simulink model "test_integration"  (R2022b)
settings: Solver=FixedStepAuto  StartTime=0.0  StopTime=240  FixedStep=0.1  RelTol=1e-3
(part 2 of 2)

== stateflow chart test_integration/Test Assessment Block ==
  state IncreasePower
    state Init
      state Verify_IP_Init
        verify(alert_led==0 && led==0 && onoff_led==0);
        settings: description=|
            | Inizializzazione.
            | Tutti i led sono spenti.
      state Verify_IP_TurnON
        verify(alert_led==0 && led==0 && onoff_led==1);
        settings: description=|
            | Accensione dispositivo.
            | Il led di accensione è acceso.
      state Verify_IP_IncreasePower300W
        verify(alert_led==0 && led==0 && onoff_led==1);
        settings: description=|
            | Richiesta di aumento potenza.
            | Il led di accensione è acceso.
      state Verify_IP_Wait300W
        verify(alert_led==0 && led==0 && onoff_led==1);
        settings: description=|
            | Attesa passaggio di potenza.
            | Il led di accensione è acceso.
      state Verify_IP_Set300W
        verify(alert_led==0 && led==1 && onoff_led==1)
        settings: description=|
            | Conferma della nuova potenza.
            | Il led di accensione è acceso ed il led giallo di attivazione sta blinkando con periodo di 2 s.
      state Verify_IP_IncreasePower500W
        verify(alert_led==0 && led==1 && onoff_led==1);
        settings: description=|
            | Richiesta di ulteriore incremento della potenza.
            | Il led di accensione è acceso ed il led giallo di attivazione sta blinkando con periodo di 2 s.
      state Verify_IP_Wait500W
        settings: description=Attesa del passaggio di potenza.
        state Verify__IP_Wait500W_1
          verify(alert_led==0 && led==1 && onoff_led==1);
          settings: description=led giallo di attivazione on
        state Verify_IP_Wait500W_2
          verify(alert_led==0 && led==0 && onoff_led==1);
          settings: description=led giallo di attivazione off
        state Verify_IP_Wait500W_3
          verify(alert_led==0 && led==1 && onoff_led==1);
          settings: description=|
              | led giallo di attivazione on
              | led giallo di attivazione off
        state Verify_IP_Wait500W_4
          verify(alert_led==0 && led==0 && onoff_led==1);
        (default) -> Verify__IP_Wait500W_1
        Verify__IP_Wait500W_1 -> Verify_IP_Wait500W_2 : [
            | after(2-(1+2*SamplePeriod),sec)
            | ]
        Verify_IP_Wait500W_2 -> Verify_IP_Wait500W_3 : [
            | after(2,sec)
            | ]
        Verify_IP_Wait500W_3 -> Verify_IP_Wait500W_4 : [
            | after(2,sec)
            | ]
      state Verify_IP_Set500W
        verify(alert_led==0 && led==0 && onoff_led==1)
        settings: description=|
            | Conferma della nuova potenza.
            | Il led di accensione è acceso ed il led giallo di attivazione sta blinkando con periodo di 1 s.
      state Init_1
      (default) -> (junction 144)
      IncreasePower.Init -> (junction 144)
      (junction 144) -> (junction 145) [order 1] : [Active_Step_In == ActiveStepInt.IP_Init
          | ]
      (junction 145) -> Verify_IP_Init [order 1] : [~in(IncreasePower.Init.Verify_IP_Init)]
      (junction 144) -> (junction 154) [order 2]
      (junction 145) -> (junction 148) [order 2]
      (junction 154) -> (junction 155) [order 1] : [Active_Step_In == ActiveStepInt.IP_TurnON
          | ]
      (junction 155) -> Verify_IP_TurnON [order 1] : [~in(IncreasePower.Init.Verify_IP_TurnON)]
      (junction 154) -> (junction 162) [order 2]
      (junction 155) -> (junction 158) [order 2]
      (junction 162) -> (junction 163) [order 1] : [Active_Step_In == ActiveStepInt.IP_IncreasePower300W
          | ]
      (junction 163) -> Verify_IP_IncreasePower300W [order 1] : [~in(IncreasePower.Init.Verify_IP_IncreasePower300W)]
      (junction 162) -> (junction 170) [order 2]
      (junction 163) -> (junction 166) [order 2]
      (junction 170) -> (junction 171) [order 1] : [Active_Step_In == ActiveStepInt.IP_Wait300W
          | ]
      (junction 171) -> Verify_IP_Wait300W [order 1] : [~in(IncreasePower.Init.Verify_IP_Wait300W)]
      (junction 170) -> (junction 178) [order 2]
      (junction 171) -> (junction 174) [order 2]
      (junction 178) -> (junction 179) [order 1] : [Active_Step_In == ActiveStepInt.IP_Set300W
          | ]
      (junction 179) -> Verify_IP_Set300W [order 1] : [~in(IncreasePower.Init.Verify_IP_Set300W)]
      (junction 178) -> (junction 186) [order 2]
      (junction 179) -> (junction 182) [order 2]
      (junction 186) -> (junction 187) [order 1] : [Active_Step_In == ActiveStepInt.IP_IncreasePower500W
          | ]
      (junction 187) -> Verify_IP_IncreasePower500W [order 1] : [~in(IncreasePower.Init.Verify_IP_IncreasePower500W)]
      (junction 186) -> (junction 195) [order 2]
      (junction 187) -> (junction 190) [order 2]
      (junction 195) -> (junction 196) [order 1] : [Active_Step_In == ActiveStepInt.IP_Wait500W
          | ]
      (junction 196) -> Verify_IP_Wait500W [order 1] : [~in(IncreasePower.Init.Verify_IP_Wait500W)]
      (junction 195) -> (junction 203) [order 2]
      (junction 196) -> (junction 199) [order 2]
      (junction 203) -> (junction 204) [order 1] : [Active_Step_In == ActiveStepInt.IP_Set500W
          | ]
      (junction 204) -> Verify_IP_Set500W [order 1] : [~in(IncreasePower.Init.Verify_IP_Set500W)]
      (junction 203) -> (junction 211) [order 2]
      (junction 204) -> (junction 207) [order 2]
      (junction 211) -> (junction 212)
      (junction 212) -> IncreasePower.Init.Init_1 [order 1] : [~in(IncreasePower.Init.Init_1)]
      (junction 212) -> (junction 215) [order 2]
    (default) -> IncreasePower.Init
  state DecreasePower
    state Init
      state Verify_DP_Init
        verify(alert_led==0 && led==0 && onoff_led==0);
        settings: description=|
            | Inizializzazione.
            | Tutti i led sono spenti.
      state Verify_DP_TurnON
        verify(alert_led==0 && led==0 && onoff_led==1);
        settings: description=|
            | Accensione del dispositivo.
            | Il led di accensione è acceso.
      state Verify_DP_IncreasePower300W
        verify(alert_led==0 && led==0 && onoff_led==1);
        settings: description=|
            | Richiesta di aumento della potenza.
            | Il led di accensione è acceso.
      state Verify_DP_Wait300W
        verify(alert_led==0 && led==0 && onoff_led==1);
        settings: description=|
            | Attesa del cambiamento di potenza.
            | Il led di accensione è acceso.
      state Verify_DP_Set300W
        verify(alert_led==0 && led==1 && onoff_led==1)
        settings: description=|
            | Conferma della nuova potenza.
            | Il led di accensione è acceso ed il led giallo di attivazione sta blinkando con periodo di 2 s.
      state Verify_DP_DecreasePower0W
        verify(alert_led==0 && led==1 && onoff_led==1);
        settings: description=|
            | Richiesta di decremento della potenza.
            | Il led di accensione è acceso ed il led giallo di attivazione sta blinkando con periodo di 2 s.
      state Verify_DP_Wait0W
        settings: description=Attesa del cambiamento di potenza.
        state Verify__DP_Wait0W_1
          verify(alert_led==0 && led==1 && onoff_led==1);
          settings: description=led giallo di attivazione on
        state Verify_DP_Wait0W_2
          verify(alert_led==0 && led==0 && onoff_led==1);
          settings: description=led giallo di attivazione off
        state Verify_DP_Wait0W_3
          verify(alert_led==0 && led==1 && onoff_led==1);
          settings: description=led giallo di attivazione on
        state Verify_DP_Wait0W_4
          verify(alert_led==0 && led==0 && onoff_led==1);
          settings: description=led giallo di attivazione off
        (default) -> Verify__DP_Wait0W_1
        Verify__DP_Wait0W_1 -> Verify_DP_Wait0W_2 : [
            | after(2-(1+2*SamplePeriod),sec)
            | ]
        Verify_DP_Wait0W_2 -> Verify_DP_Wait0W_3 : [
            | after(2,sec)
            | ]
        Verify_DP_Wait0W_3 -> Verify_DP_Wait0W_4 : [
            | after(2,sec)
            | ]
      state Verify_DP_Set0W
        verify(alert_led==0 && led==0 && onoff_led==1)
        settings: description=|
            | Conferma della nuova potenza di 0W.
            | Il led giallo di attivazione torna ad essere spento, mentre il verde di accensione è acceso.
      state Init_1
      DecreasePower.Init -> (junction 349)
      (default) -> (junction 349)
      (junction 349) -> (junction 350) [order 1] : [Active_Step_In == ActiveStepInt.DP_Init
          | ]
      (junction 350) -> Verify_DP_Init [order 1] : [~in(DecreasePower.Init.Verify_DP_Init)]
      (junction 349) -> (junction 359) [order 2]
      (junction 350) -> (junction 353) [order 2]
      (junction 359) -> (junction 360) [order 1] : [Active_Step_In == ActiveStepInt.DP_TurnON
          | ]
      (junction 360) -> Verify_DP_TurnON [order 1] : [~in(DecreasePower.Init.Verify_DP_TurnON)]
      (junction 359) -> (junction 367) [order 2]
      (junction 360) -> (junction 363) [order 2]
      (junction 367) -> (junction 368) [order 1] : [Active_Step_In == ActiveStepInt.DP_IncreasePower300W
          | ]
      (junction 368) -> Verify_DP_IncreasePower300W [order 1] : [~in(DecreasePower.Init.Verify_DP_IncreasePower300W)]
      (junction 367) -> (junction 375) [order 2]
      (junction 368) -> (junction 371) [order 2]
      (junction 375) -> (junction 376) [order 1] : [Active_Step_In == ActiveStepInt.DP_Wait300W
          | ]
      (junction 376) -> Verify_DP_Wait300W [order 1] : [~in(DecreasePower.Init.Verify_DP_Wait300W)]
      (junction 375) -> (junction 383) [order 2]
      (junction 376) -> (junction 379) [order 2]
      (junction 383) -> (junction 384) [order 1] : [Active_Step_In == ActiveStepInt.DP_Set300W
          | ]
      (junction 384) -> Verify_DP_Set300W [order 1] : [~in(DecreasePower.Init.Verify_DP_Set300W)]
      (junction 383) -> (junction 391) [order 2]
      (junction 384) -> (junction 387) [order 2]
      (junction 391) -> (junction 392) [order 1] : [Active_Step_In == ActiveStepInt.DP_DecreasePower0W
          | ]
      (junction 392) -> Verify_DP_DecreasePower0W [order 1] : [~in(DecreasePower.Init.Verify_DP_DecreasePower0W)]
      (junction 391) -> (junction 399) [order 2]
      (junction 392) -> (junction 395) [order 2]
      (junction 399) -> (junction 400) [order 1] : [Active_Step_In == ActiveStepInt.DP_Wait0W
          | ]
      (junction 400) -> Verify_DP_Wait0W [order 1] : [~in(DecreasePower.Init.Verify_DP_Wait0W)]
      (junction 399) -> (junction 416) [order 2]
      (junction 400) -> (junction 403) [order 2]
      (junction 416) -> (junction 417) [order 1] : [Active_Step_In == ActiveStepInt.DP_Set0W
          | ]
      (junction 417) -> Verify_DP_Set0W [order 1] : [~in(DecreasePower.Init.Verify_DP_Set0W)]
      (junction 417) -> (junction 420) [order 2]
      (junction 424) -> (junction 425)
      (junction 425) -> DecreasePower.Init.Init_1 [order 1] : [~in(DecreasePower.Init.Init_1)]
      (junction 425) -> (junction 428) [order 2]
      (junction 416) -> (junction 424) [order 2]
    (default) -> DecreasePower.Init
  state TurnOnOff
    state Init
      state Verify_TO_Init
        verify(alert_led==0 && led==0 && onoff_led==0);
        settings: description=|
            | Fase di inizializzazione.
            | Tutti i led sono spenti.
      state Verify_TO_PowerOn
        verify(alert_led==0 && led==0 && onoff_led==1);
        settings: description=|
            | Accensione del fornello.
            | Il led di accensione è acceso.
      state Verify_TO_Release
        verify(alert_led==0 && led==0 && onoff_led==1);
        settings: description=|
            | Rilascio del bottone
            | Il led di accensione è acceso.
      state Verify_TO_PowerOff
        verify(alert_led==0 && led==0 && onoff_led==1);
        settings: description=|
            | Pressione del bottone per lo spegnimento.
            | Il led di accensione è acceso.
      state Verify_TO_End
        state Verify_TO_End_1
          verify(alert_led==0 && led==0 && onoff_led==1);
          settings: description=led verde di accensione on
        state Verify_TO_End_2
          verify(alert_led==0 && led==0 && onoff_led==0);
          settings: description=led verde di accensione off
        (default) -> Verify_TO_End_1
        Verify_TO_End_1 -> Verify_TO_End_2 : [
            | true
            | ]
      state Verify_TO_step
        settings: description=Il fornello è spento e tutti i led sono spenti.
      (default) -> (junction 451)
      TurnOnOff.Init -> (junction 451)
      (junction 451) -> (junction 452) [order 1] : [Active_Step_In == ActiveStepInt.TO_Init
          | ]
      (junction 452) -> Verify_TO_Init [order 1] : [~in(TurnOnOff.Init.Verify_TO_Init)]
      (junction 451) -> (junction 461) [order 2]
      (junction 452) -> (junction 455) [order 2]
      (junction 461) -> (junction 462) [order 1] : [Active_Step_In == ActiveStepInt.TO_PowerOn
          | ]
      (junction 462) -> Verify_TO_PowerOn [order 1] : [~in(TurnOnOff.Init.Verify_TO_PowerOn)]
      (junction 461) -> (junction 479) [order 2]
      (junction 462) -> (junction 465) [order 2]
      (junction 479) -> (junction 480) [order 1] : [Active_Step_In == ActiveStepInt.TO_Release
          | ]
      (junction 480) -> Verify_TO_Release [order 1] : [~in(TurnOnOff.Init.Verify_TO_Release)]
      (junction 479) -> (junction 469) [order 2]
      (junction 480) -> (junction 483) [order 2]
      (junction 469) -> (junction 470) [order 1] : [Active_Step_In == ActiveStepInt.TO_PowerOff
          | ]
      (junction 470) -> Verify_TO_PowerOff [order 1] : [~in(TurnOnOff.Init.Verify_TO_PowerOff)]
      (junction 469) -> (junction 487) [order 2]
      (junction 470) -> (junction 473) [order 2]
      (junction 487) -> (junction 488) [order 1] : [Active_Step_In == ActiveStepInt.TO_End
          | ]
      (junction 488) -> Verify_TO_End [order 1] : [~in(TurnOnOff.Init.Verify_TO_End)]
      (junction 487) -> (junction 891) [order 2]
      (junction 488) -> (junction 491) [order 2]
      (junction 891) -> (junction 892)
      (junction 892) -> Verify_TO_step [order 1] : [~in(TurnOnOff.Init.Verify_TO_step)]
      (junction 892) -> (junction 895) [order 2]
    (default) -> TurnOnOff.Init
  state PotRemovedWhileCooking
    state Init
      state Verify_PR_Init_1
        verify(alert_led==0 && led==0 && onoff_led==0);
        settings: description=|
            | Inizializzazione.
            | Tutti i led sono spenti.
      state Verify_PR_TurnOn
        verify(alert_led==0 && led==0 && onoff_led==1);
        settings: description=|
            | Accensione del dispositivo.
            | Il led verde di accensione è acceso.
      state Verify_PR_IncreasePower300W
        verify(alert_led==0 && led==0 && onoff_led==1);
        settings: description=|
            | Richiesta di aumento della potenza.
            | Il led verde di accensione è acceso.
      state Verify_PR_Wait300W
        verify(alert_led==0 && led==0 && onoff_led==1);
        settings: description=|
            | Attesa del cambiamento della potenza.
            | Il led verde di accensione è acceso.
      state Verify_PR_Set300W
        verify(alert_led==0 && led==1 && onoff_led==1);
        settings: description=|
            | Conferma della nuova potenza.
            | Il led di accensione è acceso ed il led giallo di attivazione sta blinkando con periodo di 2 s.
      state Verify_PR_PotRemoved
        verify(alert_led==1 && led==1 && onoff_led==1);
        settings: description=|
            | Rimozione della pentola.
            | Il led di accensione è acceso ed il led giallo di attivazione sta blinkando con periodo di 2 s.
            | Il led rosso di allarme è acceso.
      state Verify_PR_Alarm1
        verify(alert_led==1 && led==1 && onoff_led==1);
        settings: description=|
            | Stato di allarme.
            | Il led di accensione è acceso ed il led giallo di attivazione sta blinkando con periodo di 2 s.
            | Il led rosso di allarme è acceso.
      state Verify_PR_PotPositioned
        verify(alert_led==0 && led == 1 && onoff_led==1);
        settings: description=|
            | Riposizionamento della pentola e cessazione dello stato di allarme.
            | Il led di accensione è acceso ed il led giallo di attivazione sta blinkando con periodo di 2 s.
            | Il led rosso di allarme è spento.
      state Verify_PR_ContinueWorking
        settings: description=|
            | Normale funzionamento del fornello.
            | Il led di accensione è acceso ed il led giallo di attivazione sta blinkando con periodo di 2 s.
        state Verify_PR_ContinueWorking_1
          verify(alert_led==0 && led == 1 && onoff_led==1);
          settings: description=led giallo di attivazione on
        state Verify_PR_ContinueWorking_2
          verify(alert_led==0 && led == 0 && onoff_led==1);
          settings: description=led giallo di attivazion off
        (default) -> Verify_PR_ContinueWorking_1
        Verify_PR_ContinueWorking_1 -> Verify_PR_ContinueWorking_2 : [
            | after(0.7,sec)
            | ]
      state Verify_PR_PotRemoved2
        verify(alert_led==1 && led==0 && onoff_led==1);
        settings: description=|
            | Nuova rimozione della pentola.
            | Il led di accensione è acceso ed il led giallo di attivazione sta blinkando con periodo di 2 s.
            | Il led rosso di allarme è acceso.
      state Verify_PR_Alarm2
        settings: description=|
            | Stato di allarme.
            | Il led di accensione è acceso ed il led giallo di attivazione sta blinkando con periodo di 2 s.
            | Il led rosso di allarme è acceso.
        state Verify_PR_Alarm2_1
          verify(alert_led==1 && led==0 && onoff_led==1);
          settings: description=led giallo di attivazione off
        state Verify_PR_Alarm2_2
          verify(alert_led==1 && led==1 && onoff_led==1);
          settings: description=led giallo di attivazione on
        state Verify_PR_Alarm2_3
          verify(alert_led==1 && led==0 && onoff_led==1);
          settings: description=led giallo di attivazione off
        state Verify_PR_Alarm2_4
          verify(alert_led==1 && led==1 && onoff_led==1);
          settings: description=led giallo di attivazione on
        state Verify_PR_Alarm2_5
          verify(alert_led==1 && led==0 && onoff_led==1);
          settings: description=led giallo di attivazione off
        state Verify_PR_Alarm2_6
          verify(alert_led==1 && led==1 && onoff_led==1);
          settings: description=led giallo di attivazione on
        (default) -> Verify_PR_Alarm2_1
        Verify_PR_Alarm2_1 -> Verify_PR_Alarm2_2 : [
            | after(1.8-SamplePeriod,sec)
            | ]
        Verify_PR_Alarm2_2 -> Verify_PR_Alarm2_3 : [
            | after(2,sec)
            | ]
        Verify_PR_Alarm2_3 -> Verify_PR_Alarm2_4 : [
            | after(2,sec)
            | ]
        Verify_PR_Alarm2_4 -> Verify_PR_Alarm2_5 : [
            | after(2,sec)
            | ]
        Verify_PR_Alarm2_5 -> Verify_PR_Alarm2_6 : [
            | after(2,sec)
            | ]
      state Verify_PR_TimeElapsed
        settings: description=Tempo di allarme trascorso, disattivazione del dispositivo (non eroga più potenza).
        state Verify_PR_TimeElapsed_1
          verify(alert_led==1 && led==1 && onoff_led==1);
          settings: description=|
              | led giallo di attivazione on
              | led rosso di allarme on
        state Verify_PR_TimeElapsed_2
          verify(alert_led==0 && led==0 && onoff_led==1);
          settings: description=|
              | led giallo di attivazione off
              | led rosso di allarme off
        (default) -> Verify_PR_TimeElapsed_1
        Verify_PR_TimeElapsed_1 -> Verify_PR_TimeElapsed_2 : [
            | true
            | ]
      state End_PR
        settings: description=Fornello acceso, ma non attivo, è acceso solo il led verde di accensione.
      (junction 634) -> (junction 637) [order 2]
      (junction 624) -> (junction 633) [order 2]
      (default) -> (junction 529)
      PotRemovedWhileCooking.Init -> (junction 529)
      (junction 529) -> (junction 530) [order 1] : [Active_Step_In == ActiveStepInt.PR_Init
          | ]
      (junction 530) -> Verify_PR_Init_1 [order 1] : [~in(PotRemovedWhileCooking.Init.Verify_PR_Init_1)]
      (junction 529) -> (junction 539) [order 2]
      (junction 530) -> (junction 533) [order 2]
      (junction 539) -> (junction 540) [order 1] : [Active_Step_In == ActiveStepInt.PR_TurnOn
          | ]
      (junction 540) -> Verify_PR_TurnOn [order 1] : [~in(PotRemovedWhileCooking.Init.Verify_PR_TurnOn)]
      (junction 539) -> (junction 547) [order 2]
      (junction 540) -> (junction 543) [order 2]
      (junction 547) -> (junction 548) [order 1] : [Active_Step_In == ActiveStepInt.PR_IncreasePower300W
          | ]
      (junction 548) -> Verify_PR_IncreasePower300W [order 1] : [~in(PotRemovedWhileCooking.Init.Verify_PR_IncreasePower300W)]
      (junction 547) -> (junction 555) [order 2]
      (junction 548) -> (junction 551) [order 2]
      (junction 555) -> (junction 556) [order 1] : [Active_Step_In == ActiveStepInt.PR_Wait300W
          | ]
      (junction 556) -> Verify_PR_Wait300W [order 1] : [~in(PotRemovedWhileCooking.Init.Verify_PR_Wait300W)]
      (junction 555) -> (junction 563) [order 2]
      (junction 556) -> (junction 559) [order 2]
      (junction 563) -> (junction 564) [order 1] : [Active_Step_In == ActiveStepInt.PR_Set300W
          | ]
      (junction 564) -> Verify_PR_Set300W [order 1] : [~in(PotRemovedWhileCooking.Init.Verify_PR_Set300W)]
      (junction 563) -> (junction 571) [order 2]
      (junction 564) -> (junction 567) [order 2]
      (junction 571) -> (junction 572) [order 1] : [Active_Step_In == ActiveStepInt.PR_PotRemoved
          | ]
      (junction 572) -> Verify_PR_PotRemoved [order 1] : [~in(PotRemovedWhileCooking.Init.Verify_PR_PotRemoved)]
      (junction 571) -> (junction 588) [order 2]
      (junction 572) -> (junction 575) [order 2]
      (junction 588) -> (junction 589) [order 1] : [Active_Step_In == ActiveStepInt.PR_Alarm1
          | ]
      (junction 589) -> Verify_PR_Alarm1 [order 1] : [~in(PotRemovedWhileCooking.Init.Verify_PR_Alarm1)]
      (junction 588) -> (junction 597) [order 2]
      (junction 589) -> (junction 592) [order 2]
      (junction 597) -> (junction 598) [order 1] : [Active_Step_In == ActiveStepInt.PR_PotPositioned
          | ]
      (junction 598) -> Verify_PR_PotPositioned [order 1] : [~in(PotRemovedWhileCooking.Init.Verify_PR_PotPositioned)]
      (junction 597) -> (junction 606) [order 2]
      (junction 598) -> (junction 601) [order 2]
      (junction 606) -> (junction 607) [order 1] : [Active_Step_In == ActiveStepInt.PR_ContinueWorking
          | ]
      (junction 607) -> Verify_PR_ContinueWorking [order 1] : [~in(PotRemovedWhileCooking.Init.Verify_PR_ContinueWorking)]
      (junction 606) -> (junction 615) [order 2]
      (junction 607) -> (junction 610) [order 2]
      (junction 615) -> (junction 616) [order 1] : [Active_Step_In == ActiveStepInt.PR_PotRemoved2
          | ]
      (junction 616) -> Verify_PR_PotRemoved2 [order 1] : [~in(PotRemovedWhileCooking.Init.Verify_PR_PotRemoved2)]
      (junction 615) -> (junction 624) [order 2]
      (junction 616) -> (junction 619) [order 2]
      (junction 624) -> (junction 625) [order 1] : [Active_Step_In == ActiveStepInt.PR_Alarm2
          | ]
      (junction 625) -> Verify_PR_Alarm2 [order 1] : [~in(PotRemovedWhileCooking.Init.Verify_PR_Alarm2)]
      (junction 633) -> (junction 579) [order 2]
      (junction 625) -> (junction 628) [order 2]
      (junction 633) -> (junction 634) [order 1] : [Active_Step_In == ActiveStepInt.PR_TimeElapsed
          | ]
      (junction 634) -> Verify_PR_TimeElapsed [order 1] : [~in(PotRemovedWhileCooking.Init.Verify_PR_TimeElapsed)]
      (junction 579) -> (junction 580)
      (junction 580) -> End_PR [order 1] : [~in(PotRemovedWhileCooking.Init.End_PR)]
      (junction 580) -> (junction 583) [order 2]
    (default) -> PotRemovedWhileCooking.Init
  state IncreaseAndDecreaseBothPressed
    state Init
      state Verify_BP_Init
        verify(alert_led==0 && led==0 && onoff_led==0);
        settings: description=|
            | Inizializzazione.
            | Tutti i led sono spenti.
      state Verify_BP_TurnOn
        verify(alert_led==0 && led==0 && onoff_led==1);
        settings: description=|
            | Accensione del dispositivo.
            | Il led verde di accensione è acceso.
      state Verify_BP_IncreasePower300W
        verify(alert_led==0 && led==0 && onoff_led==1);
        settings: description=|
            | Richiesta di aumento della potenza.
            | Il led verde di accensione è acceso.
      state Verify_BP_Wait300W
        verify(alert_led==0 && led==0 && onoff_led==1);
        settings: description=|
            | Attesa prima dell'effettivo cambiamento della potenza.
            | Il led verde di accensione è acceso.
      state Verify_BP_Set300W
        verify(alert_led==0 && led==1 && onoff_led==1);
        settings: description=|
            | Cambiamento della potenza.
            | Il led di accensione è acceso ed il led giallo di attivazione sta blinkando con periodo di 2 s
      state Verify_BP_BothButtonsPressed
        verify(alert_led==0 && led==1 && onoff_led==1)
        settings: description=|
            | Vengono premuti in contemporanea i bottoni di incremento e decremento della potenza.
            | Il led di accensione è acceso ed il led giallo di attivazione sta blinkando con periodo di 2 s
      state Verify_BP_ButtonsReleased
        settings: description=I bottoni vengono rilasciati. Il decremento ha la priorità.
        state Verify_BP_ButtonsReleased_1
          verify(alert_led==0 && led==1 && onoff_led==1);
          settings: description=led giallo di accensione on
        state Verify_BP_ButtonsReleased_2
          verify(alert_led==0 && led==0 && onoff_led==1);
          settings: description=led giallo di accensione off
        state Verify_BP_ButtonsReleased_3
          verify(alert_led==0 && led==1 && onoff_led==1);
          settings: description=led giallo di accensione on
        state Verify_BP_ButtonsReleased_4
          verify(alert_led==0 && led==0 && onoff_led==1);
          settings: description=led giallo di accensione off
        (default) -> Verify_BP_ButtonsReleased_1
        Verify_BP_ButtonsReleased_1 -> Verify_BP_ButtonsReleased_2 : [
            | after(2-(1+2*SamplePeriod),sec)
            | ]
        Verify_BP_ButtonsReleased_2 -> Verify_BP_ButtonsReleased_3 : [
            | after(2,sec)
            | ]
        Verify_BP_ButtonsReleased_3 -> Verify_BP_ButtonsReleased_4 : [
            | after(2,sec)
            | ]
      state Verify_BP_SetNewPower
        verify(alert_led==0 && led==0 && onoff_led==1)
        settings: description=|
            | Cambiamento di potenza effettuato.
            | La potenza attuale è 0W, il dispositivo è acceso,
            | ma non attivo ed infatti tutti i led tranne il verde sono spenti.
      state Verify_BP_End
      (default) -> (junction 685)
      IncreaseAndDecreaseBothPressed.Init -> (junction 685)
      (junction 685) -> (junction 686) [order 1] : [Active_Step_In == ActiveStepInt.BP_Init
          | ]
      (junction 686) -> Verify_BP_Init [order 1] : [~in(IncreaseAndDecreaseBothPressed.Init.Verify_BP_Init)]
      (junction 685) -> (junction 697) [order 2]
      (junction 686) -> (junction 689) [order 2]
      (junction 697) -> (junction 698) [order 1] : [Active_Step_In == ActiveStepInt.BP_TurnOn
          | ]
      (junction 698) -> Verify_BP_TurnOn [order 1] : [~in(IncreaseAndDecreaseBothPressed.Init.Verify_BP_TurnOn)]
      (junction 697) -> (junction 705) [order 2]
      (junction 698) -> (junction 701) [order 2]
      (junction 705) -> (junction 706) [order 1] : [Active_Step_In == ActiveStepInt.BP_IncreasePower300W
          | ]
      (junction 706) -> Verify_BP_IncreasePower300W [order 1] : [~in(IncreaseAndDecreaseBothPressed.Init.Verify_BP_IncreasePower300W)]
      (junction 705) -> (junction 713) [order 2]
      (junction 706) -> (junction 709) [order 2]
      (junction 713) -> (junction 714) [order 1] : [Active_Step_In == ActiveStepInt.BP_Wait300W
          | ]
      (junction 714) -> Verify_BP_Wait300W [order 1] : [~in(IncreaseAndDecreaseBothPressed.Init.Verify_BP_Wait300W)]
      (junction 713) -> (junction 721) [order 2]
      (junction 714) -> (junction 717) [order 2]
      (junction 721) -> (junction 722) [order 1] : [Active_Step_In == ActiveStepInt.BP_Set300W
          | ]
      (junction 722) -> Verify_BP_Set300W [order 1] : [~in(IncreaseAndDecreaseBothPressed.Init.Verify_BP_Set300W)]
      (junction 721) -> (junction 729) [order 2]
      (junction 722) -> (junction 725) [order 2]
      (junction 729) -> (junction 730) [order 1] : [Active_Step_In == ActiveStepInt.BP_BothButtonsPressed
          | ]
      (junction 730) -> Verify_BP_BothButtonsPressed [order 1] : [~in(IncreaseAndDecreaseBothPressed.Init.Verify_BP_BothButtonsPressed)]
      (junction 729) -> (junction 737) [order 2]
      (junction 730) -> (junction 733) [order 2]
      (junction 737) -> (junction 738) [order 1] : [Active_Step_In == ActiveStepInt.BP_ButtonsReleased
          | ]
      (junction 738) -> Verify_BP_ButtonsReleased [order 1] : [~in(IncreaseAndDecreaseBothPressed.Init.Verify_BP_ButtonsReleased)]
      (junction 737) -> (junction 754) [order 2]
      (junction 738) -> (junction 741) [order 2]
      (junction 754) -> (junction 755) [order 1] : [Active_Step_In == ActiveStepInt.BP_SetNewPower
          | ]
      (junction 755) -> Verify_BP_SetNewPower [order 1] : [~in(IncreaseAndDecreaseBothPressed.Init.Verify_BP_SetNewPower)]
      (junction 754) -> (junction 745) [order 2]
      (junction 755) -> (junction 758) [order 2]
      (junction 745) -> (junction 746)
      (junction 746) -> Verify_BP_End [order 1] : [~in(IncreaseAndDecreaseBothPressed.Init.Verify_BP_End)]
      (junction 746) -> (junction 749) [order 2]
    (default) -> IncreaseAndDecreaseBothPressed.Init
  state ChangePowerWhileWaiting
    state Init
      state Verify_CP_Init
        verify(alert_led==0 && led==0 && onoff_led==0);
        settings: description=|
            | Inizializzazione.
            | Tutti i led sono spenti.
      state Verify_CP_TurnON
        verify(alert_led==0 && led==0 && onoff_led==1);
        settings: description=|
            | Accensione del dispositivo.
            | Il led verde di accensione è acceso.
      state Verify_CP_IncreasePower300W
        verify(alert_led==0 && led==0 && onoff_led==1);
        settings: description=|
            | Richiesta di aumento della potenza.
            | Il led verde di accensione è acceso.
      state Verify_CP_Wait300W
        verify(alert_led==0 && led==0 && onoff_led==1);
        settings: description=|
            | Attesa di cambiamento della potenza.
            | Il led verde di accensione è acceso.
      state Verify_CP_IncreasePower500W
        verify(alert_led==0 && led==0 && onoff_led==1);
        settings: description=|
            | Nuova richiesta di aumento della potenza.
            | Il led verde di accensione è acceso.
      state Verify_CP_Wait500W
        verify(alert_led==0 && led==0 && onoff_led==1);
        settings: description=|
            | Attesa di cambiamento della potenza.
            | Il led verde di accensione è acceso.
      state Verify_CP_Set500W
        verify(alert_led==0 && led==1 && onoff_led==1)
        settings: description=|
            | Conferma della nuova potenza selezionata.
            | Il led di accensione è acceso ed il led giallo di attivazione sta blinkando con periodo di 1 s
      state Verify_CP_end
      (default) -> (junction 799)
      ChangePowerWhileWaiting.Init -> (junction 799)
      (junction 799) -> (junction 800) [order 1] : [Active_Step_In == ActiveStepInt.CP_Init
          | ]
      (junction 800) -> Verify_CP_Init [order 1] : [~in(ChangePowerWhileWaiting.Init.Verify_CP_Init)]
      (junction 799) -> (junction 808) [order 2]
      (junction 800) -> (junction 803) [order 2]
      (junction 808) -> (junction 809) [order 1] : [Active_Step_In == ActiveStepInt.CP_TurnON
          | ]
      (junction 809) -> Verify_CP_TurnON [order 1] : [~in(ChangePowerWhileWaiting.Init.Verify_CP_TurnON)]
      (junction 808) -> (junction 816) [order 2]
      (junction 809) -> (junction 812) [order 2]
      (junction 816) -> (junction 817) [order 1] : [Active_Step_In == ActiveStepInt.CP_IncreasePower300W
          | ]
      (junction 817) -> Verify_CP_IncreasePower300W [order 1] : [~in(ChangePowerWhileWaiting.Init.Verify_CP_IncreasePower300W)]
      (junction 816) -> (junction 825) [order 2]
      (junction 817) -> (junction 820) [order 2]
      (junction 825) -> (junction 826) [order 1] : [Active_Step_In == ActiveStepInt.CP_Wait300W
          | ]
      (junction 826) -> Verify_CP_Wait300W [order 1] : [~in(ChangePowerWhileWaiting.Init.Verify_CP_Wait300W)]
      (junction 825) -> (junction 833) [order 2]
      (junction 826) -> (junction 829) [order 2]
      (junction 833) -> (junction 834) [order 1] : [Active_Step_In == ActiveStepInt.CP_IncreasePower500W
          | ]
      (junction 834) -> Verify_CP_IncreasePower500W [order 1] : [~in(ChangePowerWhileWaiting.Init.Verify_CP_IncreasePower500W)]
      (junction 833) -> (junction 841) [order 2]
      (junction 834) -> (junction 837) [order 2]
      (junction 841) -> (junction 842) [order 1] : [Active_Step_In == ActiveStepInt.CP_Wait500W
          | ]
      (junction 842) -> Verify_CP_Wait500W [order 1] : [~in(ChangePowerWhileWaiting.Init.Verify_CP_Wait500W)]
      (junction 841) -> (junction 849) [order 2]
      (junction 842) -> (junction 845) [order 2]
      (junction 849) -> (junction 850) [order 1] : [Active_Step_In == ActiveStepInt.CP_Set500W
          | ]
      (junction 850) -> Verify_CP_Set500W [order 1] : [~in(ChangePowerWhileWaiting.Init.Verify_CP_Set500W)]
      (junction 849) -> (junction 857) [order 2]
      (junction 850) -> (junction 853) [order 2]
      (junction 857) -> (junction 858)
      (junction 858) -> Verify_CP_end [order 1] : [~in(ChangePowerWhileWaiting.Init.Verify_CP_end)]
      (junction 858) -> (junction 861) [order 2]
    (default) -> ChangePowerWhileWaiting.Init
  (default) -> IncreasePower [order 1] : [Active_Scenario_Index == 1]
  (default) -> DecreasePower [order 2] : [Active_Scenario_Index == 2]
  (default) -> TurnOnOff [order 3] : [Active_Scenario_Index == 3]
  (default) -> PotRemovedWhileCooking [order 4] : [Active_Scenario_Index == 4]
  (default) -> IncreaseAndDecreaseBothPressed [order 5] : [Active_Scenario_Index == 5]
  (default) -> ChangePowerWhileWaiting [order 6] : {assert(Active_Scenario_Index == 6,'The value of Scenario Parameter ''Active_Scenario_Index'' is not valid. Use the index of the scenario to specify it.')}
  data: alert_led input boolean size=[1]; led input boolean size=[1]; onoff_led input boolean size=[1]; Active_Step_In input; Active_Scenario_Index parameter =4; SamplePeriod constant double =str2num(get_param('InductionCooker','FixedStep'))
